simulink model "sampleModel1894_sub"  (R2023a)
settings: Solver=VariableStepAuto  StartTime=0.0  StopTime=10.0  RelTol=1e-3
libraries: hdlsllib x5, simulink x3
settings Model: Creator=user1  LastModifiedBy=user1
settings OptimizationCC: BlockReduction=off  ConditionallyExecuteInputs=off

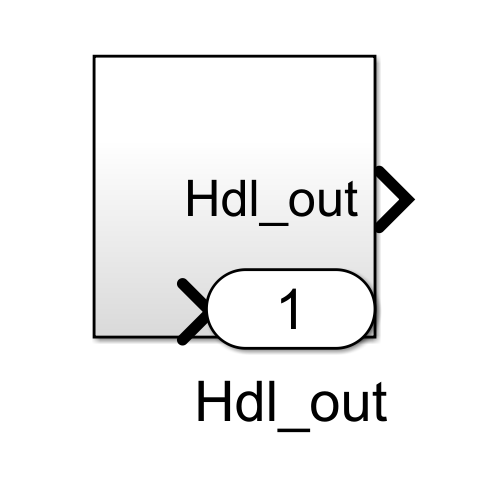
[thumbnail: Simulink's stored preview of the top-level diagram]
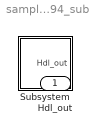
== system sampleModel1894_sub ==
  Subsystem : Subsystem
  Hdl_out : Outport  OutDataTypeStr=uint8

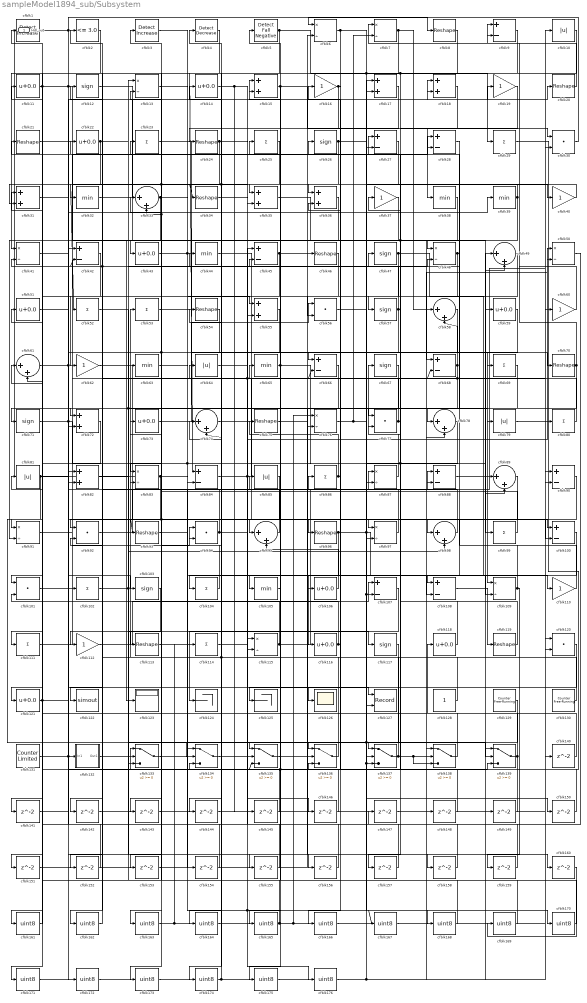
== system sampleModel1894_sub/Subsystem ==
  cfblk1 : simulink/Logic and Bit Operations/Detect Increase  vinit=0.0  OutDataTypeStr=uint8
      settings: LibrarySourceBlock=|
      | hdlsllib/Logic and Bit
      | Operations/Detect
      | Increase
  cfblk{10,64,79,81,85} (5 alike) : Abs  OutDataTypeStr=uint8  SaturateOnIntegerOverflow=off
  cfblk{9,27..28,42,45,66,68,84,88,90,100,107..108} (13 alike) : Sum  Inputs=+-  OutDataTypeStr=uint8
  cfblk{30,56,77,92,94,101,120} (7 alike) : DotProduct  OutDataTypeStr=uint8
  cfblk{23,25,29,52..53,69,80,86,99,102,104,111,114} (13 alike) : Sum  Inputs=+  OutDataTypeStr=uint8
  cfblk{12,26,47,57,67,71,103,117} (8 alike) : Signum
  cfblk{32,38..39,44,63,65,105} (7 alike) : MinMax  OutDataTypeStr=uint8
  cfblk{11,14,22,43,51,59,73,106,116,118,121} (11 alike) : Bias  Bias=0.0  SaturateOnIntegerOverflow=off
  cfblk{6..7,13,41,48,50,76,83,87,91,97,109,115} (13 alike) : Product  Inputs=*/  OutDataTypeStr=uint8  RndMeth=Zero  SaturateOnIntegerOverflow=on
  cfblk{16,19,37,40,60,62,110,112} (8 alike) : Gain  OutDataTypeStr=uint8
  cfblk{8,20..21,24,34,46,54,70,75,93,96,113,119} (13 alike) : Reshape
  cfblk122 : ToWorkspace  VariableName=simout  SaveFormat=Timeseries  SampleTime=-1
  cfblk123 : Display
  cfblk124 : Terminator
  cfblk125 : Terminator
  cfblk126 : Scope
  cfblk127 : Record  FileSettingsInternal="{\"entries\":[{\"content\":{\"excelSettings\":{\"content\":{},\"type\":\"Streamout.ExcelSettings\"}},\"type\":\"Streamout.FileSettingStorage\",\"uuid\":\"\"}],\"packageUris\":[\"http:\\/\\/schema.mathworks.com\\/mf0\\/streamout_blocks\\/R2020a\"],\"version\":\"1.0\"}"  Layout=[1 1]  SignalsInternal="{\"entries\":[{\"content\":{\"signals\":[{\"content\":{\"blockPath\":[],\"dimensions\":[1],\"domain\":\"\",\"lineColor\":\"#a2142f\",\"plots\":[1],\"port\":1,\"signalID\":49270,\"signalName\":\"cfblk31\"},\"type\":\"RecordBlkView.Signal\",\"uuid\":\"\"},{\"content\":{\"blockPath\":[],\"dimensions\":[1],\"domain\":\"\",\"lineColor\":\"#139fff\",\"plots\":[1],\"port\":2,\"signalID\":49273,\"signalName\":\"cfblk65\"},\"type\":\"RecordBlkView.Signal\",\"uuid\":\"\"}]},\"type\":\"RecordBlkView.InputSignals\",\"uuid\":\"\"}],\"packageUris\":[\"http:\\/\\/schema.mathworks.com\\/mf0\\/streamout_blocks\\/R2020a\"],\"version\":\"1.0\"}"  VisualizationBindings="{\"xyplotplugin\":{\"info\":[{\"series\":[{\"bindingParametersList\":[{\"parameter\":\"X-Axis\",\"signalID\":49270,\"signalName\":\"cfblk31\"},{\"parameter\":\"Y-Axis\",\"signalID\":49273,\"signalName\":\"cfblk65\"}],\"seriesID\":16451}],\"subplotID\":1}]}}"  CompatibilityTag=XY  st=-1
  cfblk128 : Constant  OutDataTypeStr=uint8  SampleTime=-1
  cfblk129 : hdlsllib/Sources/Counter Free-Running  NumBits=16  tsamp=-1
  cfblk130 : hdlsllib/Sources/Counter Free-Running  NumBits=16  tsamp=-1
  cfblk131 : hdlsllib/Sources/Counter Limited  uplimit=7  tsamp=-1
  cfblk132 : Subsystem
      settings: LibrarySourceBlock=|
      | hdlsllib/Ports &
      | Subsystems/Subsystem
  cfblk{133..139} (7 alike) : Switch  OutDataTypeStr=uint8  SaturateOnIntegerOverflow=off  InputSameDT=off
  cfblk{140..160} (21 alike) : Delay  SampleTime=1
  cfblk{15,17..18,31,35..36,55,72,82} (9 alike) : Sum  OutDataTypeStr=uint8
  cfblk{161..176} (16 alike) : DataTypeConversion  OutDataTypeStr=uint8  SaturateOnIntegerOverflow=off  RndMeth=Floor
  cfblk2 : hdlsllib/Logic and Bit Operations/Compare To Constant  relop=<=  const=3.0  OutDataTypeStr=uint8
  cfblk3 : simulink/Logic and Bit Operations/Detect Increase  vinit=0.0  OutDataTypeStr=uint8
      settings: LibrarySourceBlock=|
      | hdlsllib/Logic and Bit
      | Operations/Detect
      | Increase
  cfblk{33,49,58,61,74,78,89,95,98} (9 alike) : Sum  Inputs=|++  OutDataTypeStr=uint8
  cfblk4 : simulink/Logic and Bit Operations/Detect Decrease  vinit=0.0  OutDataTypeStr=uint8
      settings: LibrarySourceBlock=|
      | hdlsllib/Logic and Bit
      | Operations/Detect
      | Decrease
  cfblk5 : hdlsllib/Logic and Bit Operations/Detect Fall Negative  vinit=0  OutDataTypeStr=uint8
  Hdl_out : Outport  OutDataTypeStr=uint8
  wires:
  cfblk87/1 -> cfblk67/1
  cfblk78/1 -> cfblk97/2, cfblk104/1
  cfblk128/1 -> cfblk53/1
  cfblk38/1 -> cfblk123/1
  cfblk97/1 -> cfblk86/1
  cfblk73/1 -> cfblk56/1
  cfblk96/1 -> cfblk105/1, cfblk170/1, cfblk109/2
  cfblk52/1 -> cfblk76/2, cfblk117/1
  cfblk9/1 -> cfblk41/1
  cfblk15/1 -> cfblk30/1, cfblk125/1
  cfblk101/1 -> cfblk94/1
  cfblk36/1 -> cfblk43/1
  cfblk58/1 -> cfblk143/1, cfblk142/1
  cfblk47/1 -> cfblk136/1, cfblk110/1
  cfblk11/1 -> cfblk151/1, cfblk97/1, cfblk48/1
  cfblk8/1 -> cfblk57/1, cfblk27/2, cfblk84/1
  cfblk108/1 -> cfblk119/1
  cfblk91/1 -> cfblk64/1
  cfblk62/1 -> cfblk95/1
  cfblk29/1 -> cfblk133/1
  cfblk111/1 -> cfblk26/1
  cfblk24/1 -> cfblk66/1, cfblk101/1
  cfblk23/1 -> cfblk109/1
  cfblk46/1 -> cfblk62/1
  cfblk19/1 -> cfblk38/1
  cfblk16/1 -> cfblk106/1, cfblk24/1
  cfblk49/1 -> cfblk171/1
  cfblk7/1 -> cfblk58/1, cfblk92/1
  cfblk18/1 -> cfblk77/1
  cfblk107/1 -> cfblk124/1
  cfblk22/1 -> cfblk18/2, cfblk121/1
  cfblk39/1 -> cfblk35/1, cfblk157/1, cfblk91/2
  cfblk28/1 -> cfblk78/1
  cfblk130/1 -> cfblk63/1
  cfblk14/1 -> cfblk145/1, cfblk100/1
  cfblk5/1 -> cfblk29/1, cfblk74/2, cfblk34/1
  cfblk41/1 -> cfblk102/1
  cfblk86/1 -> cfblk126/1, cfblk5/1
  cfblk85/1 -> cfblk112/1
  cfblk12/1 -> cfblk68/1
  cfblk32/1 -> cfblk20/1
  cfblk115/1 -> cfblk73/1, cfblk10/1
  cfblk63/1 -> cfblk135/1
  cfblk43/1 -> cfblk45/2, cfblk69/1
  cfblk81/1 -> cfblk88/2, cfblk134/2
  cfblk116/1 -> cfblk166/1, cfblk11/1
  cfblk100/1 -> cfblk116/1
  cfblk70/1 -> cfblk9/2, cfblk135/2
  cfblk27/1 -> cfblk122/1
  cfblk26/1 -> cfblk40/1, cfblk52/1, cfblk113/1, cfblk93/1
  cfblk131/1 -> cfblk139/3, cfblk132/1(In1)
  cfblk106/1 -> cfblk95/2
  cfblk17/1 -> cfblk35/2
  cfblk79/1 -> cfblk50/1
  cfblk44/1 -> cfblk96/1
  cfblk83/1 -> Hdl_out/1, cfblk108/2, cfblk133/2
  cfblk54/1 -> cfblk83/1
  cfblk42/1 -> cfblk61/2
  cfblk90/1 -> cfblk174/1
  cfblk40/1 -> cfblk32/1
  cfblk30/1 -> cfblk6/1
  cfblk135/1 -> cfblk46/1
  cfblk132/1(Out1) -> cfblk48/2
  cfblk95/1 -> cfblk33/2, cfblk33/1
  cfblk134/1 -> cfblk115/2
  cfblk3/1 -> cfblk55/1
  cfblk72/1 -> cfblk111/1
  cfblk118/1 -> cfblk37/1
  cfblk33/1 -> cfblk136/2, cfblk91/1
  cfblk68/1 -> cfblk58/2, cfblk152/1, cfblk66/2
  cfblk51/1 -> cfblk98/1
  cfblk34/1 -> cfblk176/1, cfblk167/1
  cfblk37/1 -> cfblk82/2
  cfblk57/1 -> cfblk72/2, cfblk44/1, cfblk137/1
  cfblk77/1 -> cfblk47/1, cfblk16/1
  cfblk120/1 -> cfblk165/1
  cfblk35/1 -> cfblk89/1
  cfblk105/1 -> cfblk25/1
  cfblk89/1 -> cfblk108/1
  cfblk110/1 -> cfblk21/1
  cfblk136/1 -> cfblk92/2, cfblk14/1
  cfblk129/1 -> cfblk137/2, cfblk133/3
  cfblk6/1 -> cfblk100/2, cfblk36/1
  cfblk119/1 -> cfblk27/1
  cfblk109/1 -> cfblk159/1, cfblk41/2
  cfblk99/1 -> cfblk23/1
  cfblk76/1 -> cfblk7/2, cfblk17/1
  cfblk66/1 -> cfblk72/1
  cfblk4/1 -> cfblk163/1
  cfblk104/1 -> cfblk3/1
  cfblk13/1 -> cfblk168/1
  cfblk112/1 -> cfblk107/1
  cfblk60/1 -> cfblk7/1
  cfblk65/1 -> cfblk127/2, cfblk15/1
  cfblk82/1 -> cfblk65/1
  cfblk53/1 -> cfblk70/1
  cfblk92/1 -> cfblk17/2
  cfblk137/1 -> cfblk85/1, cfblk50/2, cfblk138/3
  cfblk1/1 -> cfblk8/1, cfblk103/1
  cfblk121/1 -> cfblk18/1, cfblk31/1
  cfblk74/1 -> cfblk79/1
  cfblk139/1 -> cfblk136/3, cfblk54/1
  cfblk98/1 -> cfblk83/2
  cfblk133/1 -> cfblk87/1
  cfblk71/1 -> cfblk19/1, cfblk99/1, cfblk84/2
  cfblk64/1 -> cfblk68/2, cfblk139/2
  cfblk94/1 -> cfblk88/1, cfblk12/1, cfblk42/2
  cfblk45/1 -> cfblk28/2, cfblk71/1
  cfblk21/1 -> cfblk55/2
  cfblk88/1 -> cfblk89/2
  cfblk25/1 -> cfblk31/2
  cfblk48/1 -> cfblk56/2, cfblk28/1
  cfblk20/1 -> cfblk9/1
  cfblk56/1 -> cfblk150/1, cfblk107/2
  cfblk31/1 -> cfblk127/1
  cfblk138/1 -> cfblk118/1
  cfblk80/1 -> cfblk22/1
  cfblk102/1 -> cfblk156/1, cfblk98/2
  cfblk84/1 -> cfblk80/1, cfblk60/1
  cfblk61/1 -> cfblk158/1, cfblk39/1
  cfblk140/1 -> cfblk1/1
  cfblk69/1 -> cfblk141/1
  cfblk142/1 -> cfblk138/1
  cfblk143/1 -> cfblk30/2
  cfblk67/1 -> cfblk144/1
  cfblk144/1 -> cfblk139/1
  cfblk145/1 -> cfblk115/1
  cfblk114/1 -> cfblk146/1
  cfblk146/1 -> cfblk101/2
  cfblk50/1 -> cfblk147/1
  cfblk147/1 -> cfblk78/2
  cfblk148/1 -> cfblk36/2
  cfblk149/1 -> cfblk138/2
  cfblk150/1 -> cfblk77/2
  cfblk151/1 -> cfblk6/2
  cfblk152/1 -> cfblk82/1
  cfblk117/1 -> cfblk153/1
  cfblk153/1 -> cfblk134/1
  cfblk93/1 -> cfblk154/1
  cfblk154/1 -> cfblk42/1
  cfblk113/1 -> cfblk155/1
  cfblk155/1 -> cfblk61/1
  cfblk156/1 -> cfblk15/2
  cfblk157/1 -> cfblk134/3
  cfblk158/1 -> cfblk94/2
  cfblk159/1 -> cfblk45/1
  cfblk75/1 -> cfblk160/1
  cfblk2/1 -> cfblk161/1
  cfblk161/1 -> cfblk81/1
  cfblk103/1 -> cfblk162/1
  cfblk162/1 -> cfblk2/1
  cfblk163/1 -> cfblk114/1, cfblk59/1
  cfblk55/1 -> cfblk164/1
  cfblk164/1 -> cfblk4/1
  cfblk165/1 -> cfblk51/1, cfblk76/1, cfblk149/1
  cfblk166/1 -> cfblk120/1
  cfblk167/1 -> cfblk120/2
  cfblk168/1 -> cfblk135/3, cfblk75/1
  cfblk160/1 -> cfblk169/1
  cfblk169/1 -> cfblk13/1
  cfblk170/1 -> cfblk13/2
  cfblk171/1 -> cfblk140/1, cfblk137/3, cfblk87/2
  cfblk141/1 -> cfblk172/1
  cfblk172/1 -> cfblk49/1
  cfblk10/1 -> cfblk173/1
  cfblk173/1 -> cfblk49/2
  cfblk174/1 -> cfblk74/1, cfblk148/1
  cfblk59/1 -> cfblk175/1
  cfblk175/1 -> cfblk90/1
  cfblk176/1 -> cfblk90/2

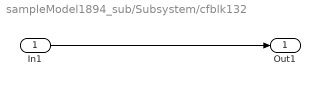
== system sampleModel1894_sub/Subsystem/cfblk132 ==
  In1 : Inport
  Out1 : Outport
  wires:
  In1/1 -> Out1/1
